simulink model "CruiseControl_pp_harness_ReqProve"  (R2015a)
settings: Solver=ode3  StartTime=0  StopTime=0.40000000000000002  FixedStep=0.10000000000000001  RelTol=1e-3
PreLoadFcn:
  | CruiseControl_dd;
undefined symbols (not defined in the file): sigbuilder_block
libraries: propertyLib x2, simulink x1, ctrlVerLib x1
settings Model: SldvGeneratedHarnessModel=TestUnitModel=CruiseControl_pp|  SnapshotInterval=1  CovMetricSettings=dcme  CovHtmlReporting=off  covSaveCumulativeToWorkspaceVar=off  CovSaveSingleToWorkspaceVar=off  CovSFcnEnable=off  Creator=The MathWorks Inc.  LastModifiedBy=colosky
settings DataIOCC: SaveFormat=StructureWithTime  SaveOutput=off  SaveTime=off
settings OptimizationCC: BlockReduction=off  InlineParams=on  InlineInvariantSignals=on  ExpressionFolding=off  ExpressionDepthLimit=2147483647  InitFltsAndDblsToZero=on
settings DebuggingCC: SaveWithParameterizedLinksMsg=none  UnderspecifiedInitializationDetection=Classic  MergeDetectMultiDrivingBlocksExec=none  SolverPrmCheckMsg=warning  InheritedTsInSrcMsg=none  FcnCallInpInsideContextMsg=UseLocalSettings  StateNameClashWarn=warning  StrictBusMsg=ErrorOnBusTreatedAsVector
settings SFSimCC: SimParseCustomCode=off
settings GRTTargetCC: TargetFcnLib=ansi_tfl_tmw.mat  CombineOutputUpdateFcns=off  GRTInterface=on
settings ConfigComp: Description=Design Verifier Custom Configuration Component  DVMode=PropertyProving  DVMaxProcessTime=3000  DVDisplayUnsatisfiableObjectives=on  DVAutomaticStubbing=off  DVMakeOutputFilesUnique=off  DVParametersUseConfig=on  DVModelCoverageObjectives=MCDC  DVMaxTestCaseSteps=500  DVTestSuiteOptimization=CombinedObjectives  DVAssertions=EnableAll  DVProofAssumptions=EnableAll  DVDetectIntegerOverflow=off  DVDetectActiveLogic=on  DVMaxViolationSteps=10  DVSaveDataFile=off  DVReportIncludeGraphics=on  DVDisplayResultsOnModel=on

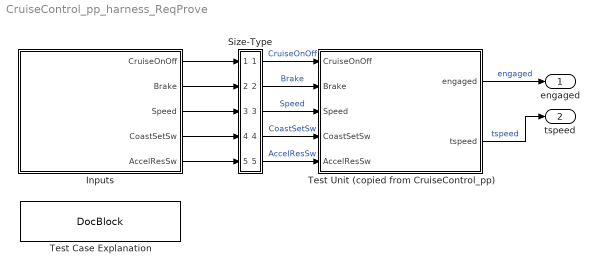
== system CruiseControl_pp_harness_ReqProve ==
  Inputs : Subsystem  Tag=STV Subsys  LoadFcn=sigbuilder_block('load',[5.4 -66.6 421.2 357.6 ]);  StartFcn=sigbuilder_block('start');  StopFcn=sigbuilder_block('stop');  ClipboardFcn=sigbuilder_block('clipboard');  mask(Sigbuilder block){}
      mask init:
      | if ~strcmp(get_param(bdroot(gcb),'SimulationStatus'),'stopped'),tuvar = sigbuilder_block('maskInit'); end
      settings: CopyFcn=sigbuilder_block('copy');  DeleteFcn=sigbuilder_block('delete');  ModelCloseFcn=sigbuilder_block('modelClose');  PreSaveFcn=sigbuilder_block('preSave');  PauseFcn=sigbuilder_block('pause');  ContinueFcn=sigbuilder_block('continue');  NameChangeFcn=sigbuilder_block('namechange');  OpenFcn=sigbuilder_block('open');  CloseFcn=sigbuilder_block('close');
      mask Display: plot(0, 0, 100, 100,[2, 2, 32, 32, 2], [68, 8, 8, 68, 68],[32, 2], [38, 38], [32, 19, 2],[53, 60, 44], [32, 17, 17, 2],[16, 16, 31, 31]);txt = getActiveGroup(gcbh);text(2, 100, txt,'verticalAlignment', 'top');
  Size-Type : Subsystem
  Test Case Explanation : simulink/Model-Wide Utilities/DocBlock  DocumentType=Text
  Test Unit (copied from CruiseControl_pp) : Subsystem
  engaged : Outport  OutDataTypeStr=boolean  PortDimensions=1
  tspeed : Outport  Port=2  OutDataTypeStr=uint8  PortDimensions=1
  wires:
  Inputs/1(CruiseOnOff) -> Size-Type/1(In1)
  Size-Type/1(Out1) -> Test Unit (copied from CruiseControl_pp)/1(CruiseOnOff)  "CruiseOnOff"
  Inputs/2(Brake) -> Size-Type/2(In2)
  Size-Type/2(Out2) -> Test Unit (copied from CruiseControl_pp)/2(Brake)  "Brake"
  Inputs/3(Speed) -> Size-Type/3(In3)
  Size-Type/3(Out3) -> Test Unit (copied from CruiseControl_pp)/3(Speed)  "Speed"
  Inputs/4(CoastSetSw) -> Size-Type/4(In4)
  Size-Type/4(Out4) -> Test Unit (copied from CruiseControl_pp)/4(CoastSetSw)  "CoastSetSw"
  Inputs/5(AccelResSw) -> Size-Type/5(In5)
  Size-Type/5(Out5) -> Test Unit (copied from CruiseControl_pp)/5(AccelResSw)  "AccelResSw"
  Test Unit (copied from CruiseControl_pp)/1(engaged) -> engaged/1  "engaged"
  Test Unit (copied from CruiseControl_pp)/2(tspeed) -> tspeed/1  "tspeed"

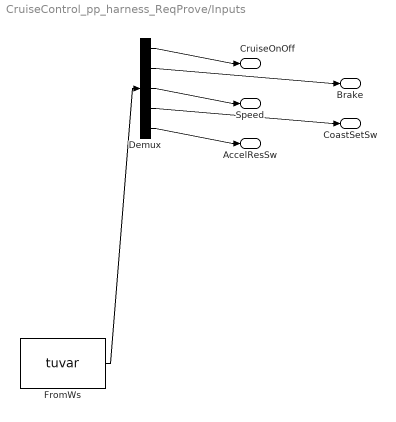
== system CruiseControl_pp_harness_ReqProve/Inputs ==
  Demux : Demux  Tag=STV Demux  Outputs=5
  FromWs : FromWorkspace  Tag=STV FromWs  VariableName=tuvar  SampleTime=0
      SigBuilderData=|
      | dataSet.timeRange = [0 0.4]
      | dataSet.name = 'Counterexample 1'
      | sbobj.Name = 'Signal Builder'
      | sbobj.Groups.Name = 'Counterexample 1'
      | sbobj.Groups.Signals(1).Name = 'CruiseOnOff'
      | sbobj.Groups.Signals(1).XData = [0 0.1 0.2 0.3 0.4]
      | sbobj.Groups.Signals(1).YData = [1 1 1 1 1]
      | sbobj.Groups.Signals(2).Name = 'Brake'
      | sbobj.Groups.Signals(2).XData = [0 0.1 0.2 0.3 0.4]
      | sbobj.Groups.Signals(2).YData = [0 0 0 0 0]
      | sbobj.Groups.Signals(3).Name = 'Speed'
      | sbobj.Groups.Signals(3).XData = [0 0.1 0.1 0.2 0.2 0.3 0.3 0.4]
      | sbobj.Groups.Signals(3).YData = [80 80 52 52 48 48 52 52]
      | sbobj.Groups.Signals(4).Name = 'CoastSetSw'
      | sbobj.Groups.Signals(4).XData = [0 0.1 0.1 0.2 0.2 0.3 0.4]
      | sbobj.Groups.Signals(4).YData = [1 1 0 0 1 1 1]
      | sbobj.Groups.Signals(5).Name = 'AccelResSw'
      | sbobj.Groups.Signals(5).XData = [0 0.1 0.2 0.2 0.3 0.3 0.4]
      | sbobj.Groups.Signals(5).YData = [1 1 1 0 0 1 1]
      | sbobj.Groups.TimeRange = [0 0.4]
  CruiseOnOff : Outport  Tag=STV Outport
  Brake : Outport  Tag=STV Outport  Port=2
  Speed : Outport  Tag=STV Outport  Port=3
  CoastSetSw : Outport  Tag=STV Outport  Port=4
  AccelResSw : Outport  Tag=STV Outport  Port=5
  wires:
  FromWs/1 -> Demux/1
  Demux/1 -> CruiseOnOff/1
  Demux/2 -> Brake/1
  Demux/3 -> Speed/1
  Demux/4 -> CoastSetSw/1
  Demux/5 -> AccelResSw/1

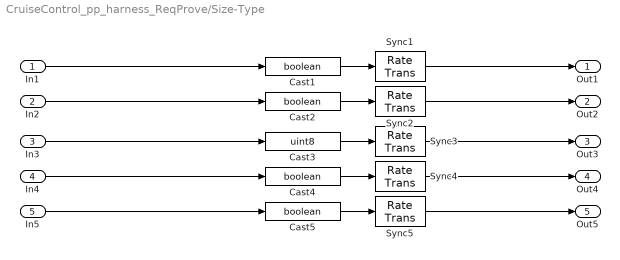
== system CruiseControl_pp_harness_ReqProve/Size-Type ==
  In1 : Inport
  In2 : Inport  Port=2
  In3 : Inport  Port=3
  In4 : Inport  Port=4
  In5 : Inport  Port=5
  Cast{1..2,4..5} (4 alike) : DataTypeConversion  OutDataTypeStr=boolean  RndMeth=Nearest  SaturateOnIntegerOverflow=on
  Cast3 : DataTypeConversion  OutDataTypeStr=uint8  RndMeth=Nearest  SaturateOnIntegerOverflow=on
  Sync{1..5} (5 alike) : RateTransition  OutPortSampleTime=[0.10000000000000001,0]
  Out1 : Outport
  Out2 : Outport  Port=2
  Out3 : Outport  Port=3
  Out4 : Outport  Port=4
  Out5 : Outport  Port=5
  wires:
  In1/1 -> Cast1/1
  Cast1/1 -> Sync1/1
  Sync1/1 -> Out1/1
  In2/1 -> Cast2/1
  Cast2/1 -> Sync2/1
  Sync2/1 -> Out2/1
  In3/1 -> Cast3/1
  Cast3/1 -> Sync3/1
  Sync3/1 -> Out3/1
  In4/1 -> Cast4/1
  Cast4/1 -> Sync4/1
  Sync4/1 -> Out4/1
  In5/1 -> Cast5/1
  Cast5/1 -> Sync5/1
  Sync5/1 -> Out5/1

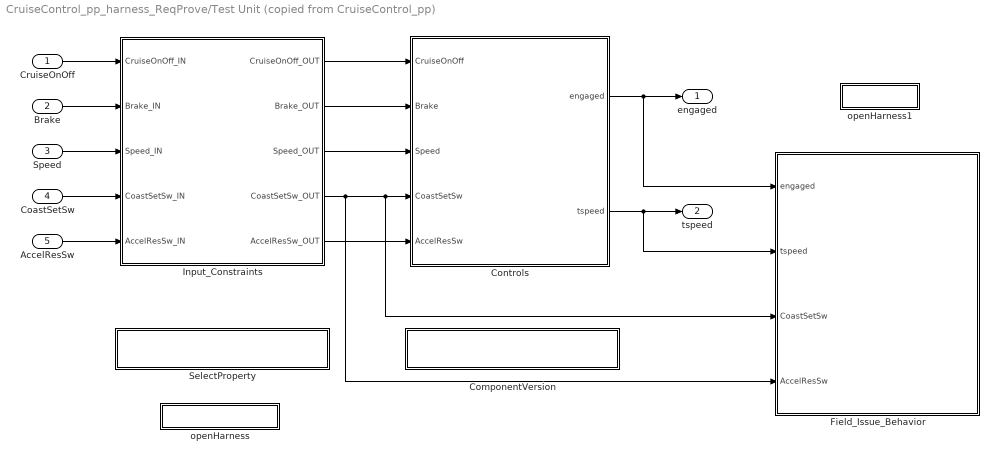
== system CruiseControl_pp_harness_ReqProve/Test Unit (copied from CruiseControl_pp) ==
  CruiseOnOff : Inport  OutDataTypeStr=boolean  PortDimensions=1
  Brake : Inport  Port=2  OutDataTypeStr=boolean  PortDimensions=1
  Speed : Inport  Port=3  OutDataTypeStr=uint8  PortDimensions=1
  CoastSetSw : Inport  Port=4  OutDataTypeStr=boolean  PortDimensions=1
  AccelResSw : Inport  Port=5  OutDataTypeStr=boolean  PortDimensions=1
  ComponentVersion : Subsystem  mask(ControlsVersion){compVer=Execution Order Sneak Fix}
      mask help: Selects the block choice for the "Controls" subystem.
      mask init:
      | compVer = get_param(gcb,'compVer');
      | compBlk = find_system(bdroot,'LookUnderMasks','on','regexp','on',...
      |     'TemplateBlock','\w+','Name','^Controls$');
      | 
      | compBlk = compBlk{1};
      | if isempty(compBlk)
      |     disp('SelectProperty:  Error! Unable to find "Controls" configurable subsystem');
      |     return;
      | end
      | switch (compVer)
      |     case 'Original'
      |         set_param(compBlk,'BlockChoice','CtrlA_Original');
      |     case 'Sneak Fix'
      |         set_param(compBlk,'BlockChoice','CtrlB_Sneak_fix');
      |     case 'Execution Order Fix'
      |         set_param(compBlk,'BlockChoice','CtrlC_ExecOrder_fix');
      |     case 'Execution Order Sneak Fix'
      |         set_param(compBlk,'BlockChoice','CtrlD_ExecOrderSneak_fix');
      |     case 'Execution Order Sneak Double Reject Fix'
      |         set_param(compBlk,'BlockChoice','CtrlE_ExecOrderSneakDblReject_fix');
      |     case 'Execution Order Limit Check Fix'
      |         set_param(compBlk,'BlockChoice','CtrlF_ExecOrderLimCheck_fix');
      |     case 'Execution Order Limit Check Sneak Fix'
      |         set_param(compBlk,'BlockChoice','CtrlG_ExecOrderLimCheckSneak_fix');
      |     case 'All Fix'
      |         set_param(compBlk,'BlockChoice','CtrlH_All_fix');
      | end
      mask TypeOptions compVer: Original | Sneak Fix | Execution Order Fix | Execution Order Sneak Fix | Execution Order Sneak Double Reject Fix | Execution Order Limit Check Fix | Execution Order Limit Check Sneak Fix | All Fix
      mask DialogControl oprnCompLib Prompt: Open Component Lib
      mask DialogControl oprnCompLib Callback:
      | close_system('ctrlVerLib');
      | open_system('ctrlVerLib');
      mask Display: disp(['Selected Version to Verify:' char(10) get_param(gcb,'compVer')]);
  Controls : Subsystem  BlockChoice=CtrlD_ExecOrderSneak_fix
      settings: AttributesFormatString=%<BlockChoice>  TemplateBlock=ctrlVerLib/ControlsCfgSub  MemberBlocks=CtrlA_Original,CtrlB_Sneak_fix,CtrlC_ExecOrder_fix,CtrlD_ExecOrderSneak_fix,CtrlE_ExecOrderSneakDblReject_fix,CtrlF_ExecOrderLimCheck_fix,CtrlG_ExecOrderLimCheckSneak_fix,CtrlH_All_fix
  Field_Issue_Behavior : Subsystem  BlockChoice=Prop_coast_minspeed
      link override Prop_accel_overspeed/Compare To Constant: const=92
      link override Prop_tspeed_LE_90/Compare To Constant: const=90
      settings: AttributesFormatString=%<BlockChoice>  TemplateBlock=propertyLib/PropertyCfgSub  MemberBlocks=Prop_accel_overspeed,Prop_coast,Prop_coast_minspeed,Prop_coast_pulse,Prop_coast_pulse_eml,Prop_none,Prop_tspeed_LE_90
  Input_Constraints : Subsystem  BlockChoice=Assum_coast_minspeed
      settings: AttributesFormatString=%<BlockChoice>  TemplateBlock=propertyLib/AssumptionCfgSub  MemberBlocks=Assum_accel_overspeed,Assum_coast,Assum_coast_minspeed,Assum_coast_pulse,Assum_coast_pulse_eml,Assum_none,Assum_tspeed_LE_90
  SelectProperty : Subsystem  mask(PropertySelection){property2prove=CoastSet with tspeed limit decrease}
      mask help: Selects the block choice for the "Input_Constraints" and "Field_Issue_Behavior" subystems.
      mask init:
      | prop = get_param(gcb,'property2prove');
      | assumpBlk = find_system(bdroot,'LookUnderMasks','on','regexp','on',...
      |     'TemplateBlock','\w+','Name',...
      |     '^Input_Constraints$');
      | %    '^Assumption');
      | 
      | assumpBlk = assumpBlk{1};
      | propBlk = find_system(bdroot,'LookUnderMasks','on','regexp','on',...
      |     'TemplateBlock','\w+','Name',...
      |     '^Field_Issue_Behavior$');
      | %    '^Property');
      |     
      | 
      | propBlk = propBlk{1};
      | if isempty(assumpBlk) || isempty(propBlk)
      |     disp('SelectProperty:  Error! Unable to find configurable subsystems');
      |     return;
      | end
      | switch (prop)
      |     case 'None'
      |         set_param(assumpBlk,'BlockChoice','Assum_none');
      |         set_param(propBlk,'BlockChoice','Prop_none');
      |     case 'tspeed<=90'
      |         set_param(assumpBlk,'BlockChoice','Assum_tspeed_LE_90');
      |         set_param(propBlk,'BlockChoice','Prop_tspeed_LE_90');
      |     case 'CoastSet with tspeed decrease'
      |         set_param(assumpBlk,'BlockChoice','Assum_coast');
      |         set_param(propBlk,'BlockChoice','Prop_coast');
      |     case 'CoastSet pulse with tspeed decrease'     
      |         set_param(assumpBlk,'BlockChoice','Assum_coast_pulse');
      |         set_param(propBlk,'BlockChoice','Prop_coast_pulse');
      |     case 'CoastSet pulse (eml) with tspeed decrease'     
      |         set_param(assumpBlk,'BlockChoice','Assum_coast_pulse_eml');
      |         set_param(propBlk,'BlockChoice','Prop_coast_pulse_eml');
      |     case 'CoastSet with tspeed limit decrease'
      |         set_param(assumpBlk,'BlockChoice','Assum_coast_minspeed');
      |         set_param(propBlk,'BlockChoice','Prop_coast_minspeed');
      |     case 'Accel overspeed'
      |         set_param(assumpBlk,'BlockChoice','Assum_accel_overspeed');
      |         set_param(propBlk,'BlockChoice','Prop_accel_overspeed');
      |     otherwise
      |         disp('SelectProperty:  Error! Unable to find configurable subsystems');
      | end
      mask TypeOptions property2prove: None | tspeed<=90 | CoastSet with tspeed decrease | CoastSet pulse with tspeed decrease | CoastSet pulse (eml) with tspeed decrease | CoastSet with tspeed limit decrease | Accel overspeed
      mask DialogControl openPropLib Prompt: Open Prop Lib
      mask DialogControl openPropLib Callback:
      | close_system('propertyLib');
      | open_system('propertyLib');
      mask Display: disp(['Selected Property to Prove:' char(10) get_param(gcb,'property2prove')]);
  openHarness : Subsystem
      settings: OpenFcn=load_PP_harness_FieldIssue;
      mask Display: disp(['Open Harness']);
  openHarness1 : Subsystem
      settings: OpenFcn=|
      | compVerSys = [bdroot '/Test Unit (copied from CruiseControl_pp)'];
      | 
      | compBlk = find_system(compVerSys,'SearchDepth',1, ...
      |     'LookUnderMasks','on','regexp','on',...
      |     'TemplateBlock','\w+','Name','^Controls$');
      | if isempty(compBlk)
      |     disp('Load Fix:  Error! Unable to find "Controls" configurable subsystem');
      |     return;
      | end
      | compBlk = compBlk{1};
      | 
      | compVerBlk = find_system(compVerSys,'SearchDepth',1,'Name','ComponentVersion');
      | if isempty(compVerBlk)
      |     disp('Load Fix:  Error! Unable to find "ComponentVersion" block');
      |     return;
      | end
      | compVerBlk = compVerBlk{1};
      | 
      | if strcmp('ReadOnly',get_param(compVerBlk,'Permissions'))
      |     return;
      | end
      | 
      | compVer = get_param(compVerBlk,'compVer');
      | switch (compVer)
      | 
      |     case 'Execution Order Fix'
      |         set_param(compVerBlk,'compVer','Execution Order Sneak Fix');
      |         set_param(compBlk,'BlockChoice','CtrlD_ExecOrderSneak_fix');
      | 
      |     case 'Execution Order Sneak Fix'
      |         set_param(compVerBlk,'compVer','Execution Order Sneak Double Reject Fix');
      |         set_param(compBlk,'BlockChoice','CtrlE_ExecOrderSneakDblReject_fix');
      | 
      |     case 'Execution Order Sneak Double Reject Fix'
      |         set_param(compVerBlk,'compVer','All Fix');
      |         set_param(compBlk,'BlockChoice','CtrlH_All_fix');
      | 
      | end
      | 
      | set_param(compVerBlk,'Permissions','ReadOnly');
      | 
      | set_param(bdroot,'SimulationCommand','Update');
      mask Display: disp('Load Fix');
  engaged : Outport  OutDataTypeStr=boolean  PortDimensions=1
  tspeed : Outport  Port=2  OutDataTypeStr=uint8  PortDimensions=1
  wires:
  Controls/2(tspeed) -> tspeed/1, Field_Issue_Behavior/2(tspeed)
  Controls/1(engaged) -> engaged/1, Field_Issue_Behavior/1(engaged)
  AccelResSw/1 -> Input_Constraints/5(AccelResSw_IN)
  Speed/1 -> Input_Constraints/3(Speed_IN)
  CruiseOnOff/1 -> Input_Constraints/1(CruiseOnOff_IN)
  Brake/1 -> Input_Constraints/2(Brake_IN)
  CoastSetSw/1 -> Input_Constraints/4(CoastSetSw_IN)
  Input_Constraints/1(CruiseOnOff_OUT) -> Controls/1(CruiseOnOff)
  Input_Constraints/2(Brake_OUT) -> Controls/2(Brake)
  Input_Constraints/3(Speed_OUT) -> Controls/3(Speed)
  Input_Constraints/4(CoastSetSw_OUT) -> Controls/4(CoastSetSw), Field_Issue_Behavior/3(CoastSetSw), Field_Issue_Behavior/4(AccelResSw)
  Input_Constraints/5(AccelResSw_OUT) -> Controls/5(AccelResSw)

== system CruiseControl_pp_harness_ReqProve/Test Unit (copied from CruiseControl_pp)/ComponentVersion ==

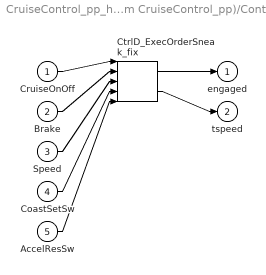
== system CruiseControl_pp_harness_ReqProve/Test Unit (copied from CruiseControl_pp)/Controls ==
  CruiseOnOff : Inport
  Brake : Inport  Port=2
  Speed : Inport  Port=3
  CoastSetSw : Inport  Port=4
  AccelResSw : Inport  Port=5
  CtrlD_ExecOrderSneak_fix : ctrlVerLib/CtrlD_ExecOrderSneak_fix
  engaged : Outport
  tspeed : Outport  Port=2
  wires:
  CruiseOnOff/1 -> CtrlD_ExecOrderSneak_fix/1
  Brake/1 -> CtrlD_ExecOrderSneak_fix/2
  Speed/1 -> CtrlD_ExecOrderSneak_fix/3
  CoastSetSw/1 -> CtrlD_ExecOrderSneak_fix/4
  AccelResSw/1 -> CtrlD_ExecOrderSneak_fix/5
  CtrlD_ExecOrderSneak_fix/1 -> engaged/1
  CtrlD_ExecOrderSneak_fix/2 -> tspeed/1

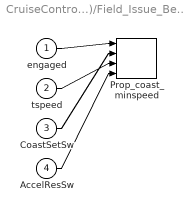
== system CruiseControl_pp_harness_ReqProve/Test Unit (copied from CruiseControl_pp)/Field_Issue_Behavior ==
  engaged : Inport
  tspeed : Inport  Port=2
  CoastSetSw : Inport  Port=3
  AccelResSw : Inport  Port=4
  Prop_coast_minspeed : propertyLib/Prop_coast_minspeed
  wires:
  engaged/1 -> Prop_coast_minspeed/1
  CoastSetSw/1 -> Prop_coast_minspeed/2
  tspeed/1 -> Prop_coast_minspeed/3
  AccelResSw/1 -> Prop_coast_minspeed/4

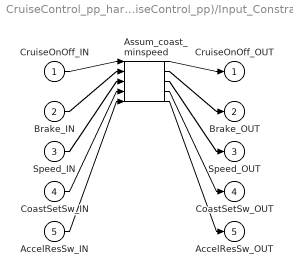
== system CruiseControl_pp_harness_ReqProve/Test Unit (copied from CruiseControl_pp)/Input_Constraints ==
  CruiseOnOff_IN : Inport
  Brake_IN : Inport  Port=2
  Speed_IN : Inport  Port=3
  CoastSetSw_IN : Inport  Port=4
  AccelResSw_IN : Inport  Port=5
  Assum_coast_minspeed : propertyLib/Assum_coast_minspeed
  CruiseOnOff_OUT : Outport
  Brake_OUT : Outport  Port=2
  Speed_OUT : Outport  Port=3
  CoastSetSw_OUT : Outport  Port=4
  AccelResSw_OUT : Outport  Port=5
  wires:
  CruiseOnOff_IN/1 -> Assum_coast_minspeed/1
  Brake_IN/1 -> Assum_coast_minspeed/2
  Speed_IN/1 -> Assum_coast_minspeed/3
  CoastSetSw_IN/1 -> Assum_coast_minspeed/4
  AccelResSw_IN/1 -> Assum_coast_minspeed/5
  Assum_coast_minspeed/1 -> CruiseOnOff_OUT/1
  Assum_coast_minspeed/2 -> Brake_OUT/1
  Assum_coast_minspeed/3 -> Speed_OUT/1
  Assum_coast_minspeed/4 -> CoastSetSw_OUT/1
  Assum_coast_minspeed/5 -> AccelResSw_OUT/1

== system CruiseControl_pp_harness_ReqProve/Test Unit (copied from CruiseControl_pp)/SelectProperty ==

== system CruiseControl_pp_harness_ReqProve/Test Unit (copied from CruiseControl_pp)/openHarness ==

== system CruiseControl_pp_harness_ReqProve/Test Unit (copied from CruiseControl_pp)/openHarness1 ==
